simulink model "Test_StrtFunc"  (R2020a)
settings: Solver=FixedStepAuto  StartTime=0.0  StopTime=10.0  FixedStep=0.1  MaxStep=0.1  RelTol=1e-3
settings Model: DataDictionary=TestConfig.sldd  Creator=toma  LastModifiedBy=toma
settings OptimizationCC: DefaultParameterBehavior=Inlined  EnhancedBackFolding=on  PassReuseOutputArgsAs=Individual arguments  ZeroExternalMemoryAtStartup=off  ZeroInternalMemoryAtStartup=off  OptimizeBlockOrder=speed  DifferentSizesBufferReuse=on  OptimizationCustomize=off  EfficientTunableParamExpr=on
settings DebuggingCC: UnderspecifiedInitializationDetection=Classic  MergeDetectMultiDrivingBlocksExec=none  ParameterTunabilityLossMsg=error  ModelReferenceSymbolNameMessage=none
settings ModelReferenceCC: PropagateSignalLabelsOutOfModel=off
settings SFSimCC: MATLABDynamicMemAlloc=off
settings RTWCC: Description=CIGRE export target  SystemTargetFile=cigre.tlc  TemplateMakefile=cigre_tmf  Toolchain=CIGRE DLL - Microsoft Visual C++ 2019 (64bit) | nmake makefile (64-bit Windows)
settings CodeAppCC: ForceParamTrailComments=on  IgnoreCustomStorageClasses=off  OperatorAnnotations=on  SimulinkDataObjDesc=on  SFDataObjDesc=on  InsertBlockDesc=on
settings STFCustomTargetCC: TargetLangStandard=C99 (ISO)  MultiwordLength=256  GenerateSampleERTMain=on  CompOptLevelCompliant=on  CombineOutputUpdateFcns=on  ERTCustomFileBanners=on  MultiInstanceERTCode=on  CodeInterfacePackaging=Reusable function  SupportContinuousTime=off  SupportNonInlinedSFcns=off  RemoveResetFunc=on  MATLABClassNameForMDSCustomization=Simulink.SoftwareTarget.ERTCustomization  UseToolchainInfoCompliant=on  SystemTargetFile=cigre.tlc
settings ERTTargetCC: TargetLangStandard=C99 (ISO)  GenerateSampleERTMain=on  ParMdlRefBuildCompliant=off  ConcurrentExecutionCompliant=off  MultiInstanceERTCode=on  CodeInterfacePackaging=Reusable function  ModelStepFunctionPrototypeControlCompliant=off  CPPClassGenCompliant=off  InlinedParameterPlacement=NonHierarchical  RootIOFormat=Structure reference  ERTCustomFileTemplate=example_file_process.tlc

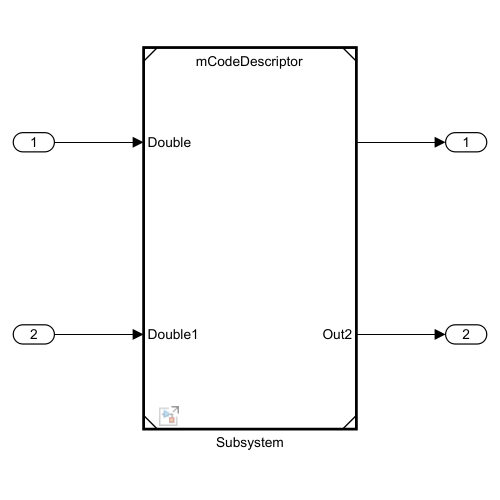
[thumbnail: Simulink's stored preview of the top-level diagram]
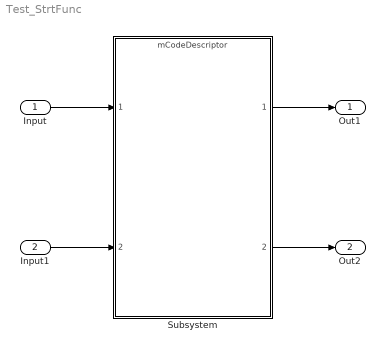
== system Test_StrtFunc ==
  Input : Inport
  Input1 : Inport  Port=2
  Subsystem : ModelReference  ModelNameDialog=mCodeDescriptor.mdl  SimulationMode=Normal  ModelReferenceVersion=20.4
  Out1 : Outport
  Out2 : Outport  Port=2
  wires:
  Input/1 -> Subsystem/1
  Subsystem/1 -> Out1/1
  Input1/1 -> Subsystem/2
  Subsystem/2 -> Out2/1
